simulink subsystem "controller_template"  (R2022a)
settings: Solver=VariableStepAuto  StartTime=0.0  StopTime=10.0  RelTol=1e-3
settings Model: Creator=humms  LastModifiedBy=Abraham
settings SolverCC: AlgebraicLoopSolver=TrustRegion
settings DebuggingCC: UnconnectedInputMsg=warning  UnconnectedOutputMsg=warning  UnconnectedLineMsg=warning  SFMachineParentedDataDiag=warning

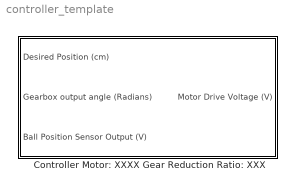
== system controller_template ==
  Controller Motor: XXXX Gear Reduction Ratio: XXX : Subsystem  Description=ECE 414 Control solution for the ball on track problem.

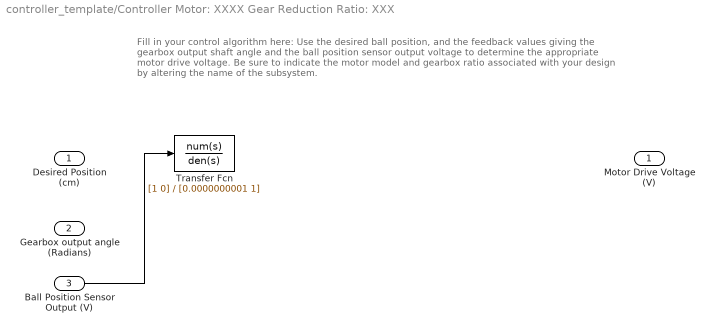
== system controller_template/Controller Motor: XXXX Gear Reduction Ratio: XXX ==
  note: Fill in your control algorithm here: Use the desired ball position, and
      | the feedback values giving the gearbox output shaft angle and the ball
      | position sensor output voltage to determine the appropriate motor drive voltage.
      |
      | Be sure to indicate the motor model and gearbox ratio associated with your
      | design by altering the name of the subsystem.
  Desired Position (cm) : Inport
  Gearbox output angle (Radians) : Inport  Port=2
  Ball Position Sensor Output (V) : Inport  Port=3
  Transfer Fcn : TransferFcn  Numerator=[1 0]  Denominator=[0.0000000001 1]
  Motor Drive Voltage (V) : Outport
  wires:
  Ball Position Sensor Output (V)/1 -> Transfer Fcn/1
